simulink model "ADPSEStaF1LCLTr"  (R2018b)
settings: Solver=ode1  StartTime=0.0  StopTime=100  FixedStep=1/1000  RelTol=1e-3  AbsTol=1e-3  EnableMultiTasking=on
PostLoadFcn:
  | f_Simulink_figureplace
InitFcn:
  | ADPSEStaF1LCLTr_PreSim
values from neighbouring files (symbols this model uses):
  ar = 3    [ADPSEStaF1LCLTr_PreSim.m]
  beta = 0.01    [ADPSEStaF1LCLTr_PreSim.m]
  etaa1 = 2    [ADPSEStaF1LCLTr_PreSim.m]
  etaa2 = 0.0010    (= 0.001)    [ADPSEStaF1LCLTr_PreSim.m]
  etac1 = 0.001    [ADPSEStaF1LCLTr_PreSim.m]
  etac2 = 2    [ADPSEStaF1LCLTr_PreSim.m]
  F = 9    [ADPSEStaF1LCLTr_PreSim.m]
  freq = unifrnd(80,100,4,100)    [ADPSEStaF1LCLTr_PreSim.m]
  fs = 1000    [ADPSEStaF1LCLTr_PreSim.m]
  Gamma0 = 50*eye(L)    [ADPSEStaF1LCLTr_PreSim.m]
  GammaTheta = 1*eye(outlayer)    [ADPSEStaF1LCLTr_PreSim.m]
  k = 500    [ADPSEStaF1LCLTr_PreSim.m]
  kTheta = M*2    (= 20)    [ADPSEStaF1LCLTr_PreSim.m]
  m = 1    [ADPSEStaF1LCLTr_PreSim.m]
  M = 10    [ADPSEStaF1LCLTr_PreSim.m]
  model = 0    [ADPSEStaF1LCLTr_PreSim.m]
  MovePoints = 1    [ADPSEStaF1LCLTr_PreSim.m]
  n = 2    [ADPSEStaF1LCLTr_PreSim.m]
  Phase = unifrnd(0,2*pi,4,100)    [ADPSEStaF1LCLTr_PreSim.m]
  Q = [10 0 ; 0 10]    [ADPSEStaF1LCLTr_PreSim.m]
  R = 1    [ADPSEStaF1LCLTr_PreSim.m]
  s = 0.7    [ADPSEStaF1LCLTr_PreSim.m]
  theta0 = 0*ones(outlayer,n)    [ADPSEStaF1LCLTr_PreSim.m]
  v = 1    [ADPSEStaF1LCLTr_PreSim.m]
  WaH0 = 0.025*ones(L,1)    [ADPSEStaF1LCLTr_PreSim.m]
  WcH0 = 0.025*ones(L,1)    [ADPSEStaF1LCLTr_PreSim.m]
  x0 = [0; 0]    [ADPSEStaF1LCLTr_PreSim.m]
undefined symbols (not defined in the file or in its folder): g, outlayer
settings Model: Creator=rkamalapurkar  LastModifiedBy=rushik
settings SolverCC: AutoScaleAbsTol=off
settings DataIOCC: SaveFormat=Array  SaveOutput=off  DSMLogging=off  SaveTime=off  SignalLoggingName=ADPSEStaF1LCLTrData
settings OptimizationCC: ExpressionDepthLimit=2147483647  LifeSpan=inf  SimCompilerOptimization=on
settings DebuggingCC: UnderspecifiedInitializationDetection=Classic  MergeDetectMultiDrivingBlocksExec=none  SolverPrmCheckMsg=warning  FcnCallInpInsideContextMsg=warning  StateNameClashWarn=warning  SFUnexpectedBacktrackingDiag=warning  SFNoUnconditionalDefaultTransitionDiag=warning  SFExecutionAtInitializationDiag=none
settings HardwareCC: ProdBitPerPointer=32  ProdBitPerSizeT=32  ProdBitPerPtrDiffT=32  ProdLargestAtomicFloat=None  ProdIntDivRoundTo=Undefined  ProdEndianess=Unspecified  ProdWordSize=32  ProdHWDeviceType=32-bit Generic
settings ModelReferenceCC: PropagateSignalLabelsOutOfModel=off
settings SFSimCC: SimUseLocalCustomCode=off
settings RTWCC: RTWUseLocalCustomCode=off
settings CodeAppCC: StateflowObjectComments=on
settings GRTTargetCC: TargetLangStandard=C89/C90 (ANSI)  GeneratePreprocessorConditionals=Disable all  CombineOutputUpdateFcns=off  GRTInterface=on
settings ConfigComp: CovMetricSettings=dw  CovHtmlReporting=on  CovSaveCumulativeToWorkspaceVar=on  CovSaveSingleToWorkspaceVar=on  CovExternalEMLEnable=off  CovSFcnEnable=off

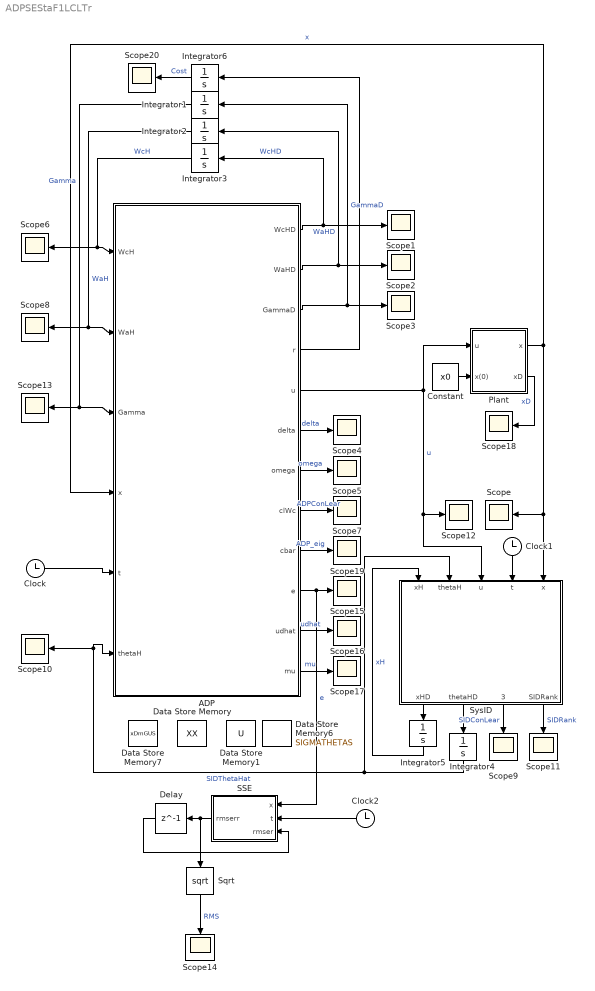
== system ADPSEStaF1LCLTr ==
  ADP : MATLAB Function  TreatAsAtomicUnit=on
  Clock : Clock
  Clock1 : Clock
  Clock2 : Clock
  Constant : Constant  Value=x0
  Data Store Memory : DataStoreMemory  DataStoreName=XX  InitialValue=zeros(n,F)  ShowAdditionalParam=off  OutDataTypeStr=double
  Data Store Memory1 : DataStoreMemory  DataStoreName=U  InitialValue=zeros(m,(F+1)/2)  ShowAdditionalParam=off  OutDataTypeStr=double
  Data Store Memory6 : DataStoreMemory  DataStoreName=SIGMATHETAS  InitialValue=zeros((outlayer),M)  ShowAdditionalParam=off  OutDataTypeStr=double
  Data Store Memory7 : DataStoreMemory  DataStoreName=xDmGUS  InitialValue=zeros(n,M)  ShowAdditionalParam=off  OutDataTypeStr=double
  Delay : Delay  DelayLength=1  InitialCondition=0
  Integrator1 : Integrator  InitialCondition=Gamma0
  Integrator2 : Integrator  InitialCondition=WaH0
  Integrator3 : Integrator  InitialCondition=WcH0
  Integrator4 : Integrator  InitialCondition=theta0
  Integrator5 : Integrator  InitialCondition=zeros(n,1)
  Integrator6 : Integrator
  Plant : Subsystem
  SSE : MATLAB Function  TreatAsAtomicUnit=on
  Scope{,1..20} (21 alike) : Scope
  Sqrt : Sqrt  SaturateOnIntegerOverflow=on
  SysID : MATLAB Function  TreatAsAtomicUnit=on
  wires:
  ADP/3(GammaD) -> Integrator1/1, Scope3/1  "GammaD"
  ADP/1(WcHD) -> Integrator3/1, Scope1/1  "WcHD"
  Integrator3/1 -> Scope6/1, ADP/1(WcH)  "WcH"
  ADP/2(WaHD) -> Integrator2/1, Scope2/1  "WaHD"
  Integrator2/1 -> Scope8/1, ADP/2(WaH)  "WaH"
  ADP/6(delta) -> Scope4/1  "delta"
  ADP/7(omega) -> Scope5/1  "omega"
  Integrator1/1 -> Scope13/1, ADP/3(Gamma)  "Gamma"
  Clock/1 -> ADP/5(t)
  ADP/5(u) -> Plant/1(u), SysID/3(u), Scope12/1  "u"
  ADP/8(clWc) -> Scope7/1  "ADPConLear"
  Integrator4/1 -> ADP/6(thetaH), Scope10/1, SysID/2(thetaH)  "SIDThetaHat"
  Plant/1(x) -> SysID/5(x), Scope/1, ADP/4(x)  "x"
  Constant/1 -> Plant/2(x(0))
  SysID/1(xHD) -> Integrator5/1
  Integrator5/1 -> SysID/1(xH)  "xH"
  SysID/4(SIDRank) -> Scope11/1  "SIDRank"
  SysID/3(SIDConLear) -> Scope9/1  "SIDConLear"
  SysID/2(thetaHD) -> Integrator4/1
  Clock1/1 -> SysID/4(t)
  ADP/10(e) -> SSE/1(x), Scope15/1  "e"
  ADP/11(udhat) -> Scope16/1  "udhat"
  ADP/12(mu) -> Scope17/1  "mu"
  Plant/2(xD) -> Scope18/1  "xD"
  ADP/9(cbar) -> Scope19/1  "ADP_eig"
  Clock2/1 -> SSE/2(t)
  SSE/1(rmserr) -> Sqrt/1, Delay/1
  Delay/1 -> SSE/3(rmser)
  Sqrt/1 -> Scope14/1  "RMS"
  ADP/4(r) -> Integrator6/1
  Integrator6/1 -> Scope20/1  "Cost"

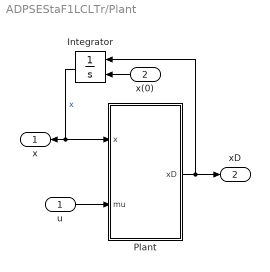
== system ADPSEStaF1LCLTr/Plant ==
  u : Inport
  x(0) : Inport  Port=2
  Integrator : Integrator  InitialConditionSource=external  InitialCondition=[1;1;0.0;0.0]
  Plant : MATLAB Function  TreatAsAtomicUnit=on
  x : Outport
  xD : Outport  Port=2
  wires:
  Plant/1(xD) -> Integrator/1, xD/1
  Integrator/1 -> Plant/1(x), x/1  "x"
  u/1 -> Plant/2(mu)
  x(0)/1 -> Integrator/2

== matlab function ADPSEStaF1LCLTr/SSE ==
  data: x input; t input; rmser input; rmserr output
function rmserr = fcn(x,t,rmser)
%#codegen

if t>90
    rmserr = rmser+(1/10000)*(norm(x))^2;
else
    rmserr = 0;
end

== matlab function ADPSEStaF1LCLTr/ADP ==
  settings: updateMethod=DISCRETE
  data: WcH input; WaH input; Gamma input; x input; t input; thetaH input; R parameter; Q parameter; etaa1 parameter; etaa2 parameter; etac1 parameter; v parameter; model parameter; WcHD output; WaHD output; GammaD output; r output; u output; delta output; omega output; clWc output; cbar output; etac2 parameter; beta parameter; n parameter; e output; udhat output; mu output; s parameter; MovePoints parameter; ar parameter; freq parameter; Phase parameter
function [WcHD,WaHD,GammaD,r,u,delta,omega,clWc,cbar,e,udhat,mu]=...
    control(WcH,WaH,Gamma,x,t,thetaH,R,Q,etaa1,etaa2,etac1,v,model,...
    etac2,beta,n,s,MovePoints,ar,freq,Phase)
%#codegen
% xd = [2*sin((1/2)*t); 2*cos((1/2)*t)+2*sin((1/2)*t)];
% if NormDyn == 1
%     a = norm(x0);
% else
%     a = 1;
% end
xd = (1/2)*[2*sin(t); 2*cos(t)+2*sin(t)];
hd = [xd(2)-xd(1); xd(2)-2*xd(1)];
e = x-xd;
Z = [e;xd];
%% Concurrent Learning
if model==1
    thetaH=[-1 -0.5; 1 0; 0 -0.5];
end
% nm=(y'*y+dbar)/(1+v2*(y'*y));
nm=1;
if MovePoints == 0
    temp=linspace(-3.0*s,3.0*s,3);
    [temp1, temp2, temp3, temp4] = ndgrid(temp,temp,temp,temp);
    XC=[temp1(:) temp2(:) temp3(:) temp4(:)]'; % matrix with columns as selected points
    N = length(temp)^(2*n); %Number of points
else
    N=1;
    XC=unifrnd(-ar*s*nm,ar*s*nm,2*n,N);
%     XC = ar*s*nm*ADPSEStaF1LCLTr_ExtTraj(t,freq,Phase);
end
clWc=zeros(size(WcH));
clWa=zeros(size(WaH));
CLmatrix=zeros(size(WcH,1),size(WcH,1));
CLGamma=zeros(size(Gamma));
parfor i=1:N
    Zi=Z+XC(:,i);
    ei=Zi(1:2,1);
    xdi=Zi(3:4,1);
    xi=ei+xdi;
    hdi = [xdi(2)-xdi(1);xdi(2)-2*xdi(1)];
    gi=[0; (cos(2*xi(1))+2)];
    gplusdi=[0 1/(cos(2*xdi(1))+2)];
    F1i = [-hdi+gi*gplusdi*hdi;hdi];
    [sigthi,~]=ADPSEStaF1LCLTr_SIDBasis(xi);
    [sigthdi,~]=ADPSEStaF1LCLTr_SIDBasis(xdi);
    Gi = [gi;zeros(size(gi))];
    [~,sig_pi,~]=ADPSEStaF1LCLTr_Basis(Zi,s,n);         
    mui=-0.5*(R\Gi')*sig_pi'*WaH;
    FTHi=[thetaH'*sigthi-gi*gplusdi*thetaH'*sigthdi;zeros(n,1)];
    omegai = sig_pi*(FTHi+F1i+Gi*mui);
%     rhoi=(1+v*omegai'*(Gamma)*omegai);
    rhoi=(1+v*(omegai'*omegai));
    ri = ei'*Q*ei + mui'*R*mui;
    deltai = WcH'*omegai + ri;
    clWc=clWc+Gamma*omegai*deltai/rhoi;
    Gsigmai = sig_pi*Gi*(R\Gi')*sig_pi';
    clWa=clWa+Gsigmai'*WaH*omegai'*WcH/(4*rhoi);
    CLmatrix=CLmatrix+omegai*omegai'/(N*rhoi);
    CLGamma=CLGamma+Gamma*(omegai*omegai'/rhoi^2)*Gamma;
end
clWc=-etac2*clWc/N;
clWa=etac2*clWa/N;
CLGamma=CLGamma/N;
cbar=real(min(svd(CLmatrix)));

%% ADP
g=[0; (cos(2*x(1))+2)];
gplusd=[0 1/(cos(2*xd(1))+2)];
F1 = [-hd+g*gplusd*hd;hd];
[sigth,~]=ADPSEStaF1LCLTr_SIDBasis(x);
[sigthd,~]=ADPSEStaF1LCLTr_SIDBasis(xd);
udhat = gplusd*(hd-thetaH'*sigthd);
G = [g;zeros(size(g))];
[~,sig_p,~]=ADPSEStaF1LCLTr_Basis(Z,s,n);         
mu=-0.5*(R\G')*sig_p'*WaH;
FTH=[thetaH'*sigth-g*gplusd*thetaH'*sigthd;zeros(n,1)];
omega = sig_p*(FTH+F1+G*mu);
Gsigma = sig_p*G*(R\G')*sig_p';
r = e'*Q*e + mu'*R*mu;
delta = WcH'*omega + r;
rho = (1+v*(omega'*omega));
WcHD = (-etac1*Gamma*omega*delta/rho+clWc);
GammaD = (beta*Gamma-Gamma*(omega*omega'/rho^2)*Gamma-CLGamma);
WaHD = etaa1*(WcH-WaH)...
    -(etaa2*WaH-etac1*Gsigma'*WaH*omega'*WcH/(4*rho))+clWa;
%% Controller
u = mu+udhat;

== matlab function ADPSEStaF1LCLTr/Plant/Plant ==
  data: xD output; x input; mu input
function xD = dynamics(x,mu)
%#codegen
F=[-x(1)+x(2) ;-0.5*x(1)-0.5*x(2)*(1-(cos(2*x(1))+2)^2)];
G=[0; (cos(2*x(1))+2)];
xD = F+G*mu;

== matlab function ADPSEStaF1LCLTr/SysID ==
  settings: updateMethod=DISCRETE
  data: xH input; xHD output; thetaH input; thetaHD output; u input; SIDConLear output; SIDRank output; t input; x input; k parameter; GammaTheta parameter; kTheta parameter; M parameter; XX data_store_memory; fs parameter; F parameter; g parameter; U data_store_memory; model parameter; SIGMATHETAS data_store_memory; xDmGUS data_store_memory
function [xHD,thetaHD,SIDConLear,SIDRank] = Control(xH,thetaH,u,t,x,k,...
    GammaTheta,kTheta,M,fs,F,g,model)
%#codegen
% This simulink block implements concurrent-learning based system
% identification using a Savitzky–Golay smoothing filter for state
% derivative computation. 
% fs: Sampling frequency
% M: number of stored data points
% F: Savitzky–Golay filter window length
% g: Savitzky–Golay filter differentiation matrix

global XX; % Data store memory for storing the values of x
global U; % Data store memory for storing the values of u
global SIGMATHETAS; % Data store for storing the values of sigth,
           % made of sigth matrices stacked in a row
global xDmGUS; % Data store memory for storing the values of xDot-G*u

%Dynamics
G=[0; (cos(2*x(1))+2)];

if model~=1
ite=round(t*fs)+1; % Current iteration number
xT = x-xH;

% Basis functions
[sigth,~]=ADPSEStaF1LCLTr_SIDBasis(x);

% At every time ite store the past F values of the state. Note that 
% Q*g(:,2)/(1/fs) gives the state derivative at ite-(F-1)/2
if ite<=F
    XX(:,ite)=x;
else
    XX = [XX(:,2:F) x];
end

% At every time ite store the past (F+1)/2 values of the control. Actually, 
% we only need the value of u at ite-(F-1)/2. However, I could not find a 
% way to store just that single value. Also, even if U is initialized as a 
% row vector, MATLAB seems to think its a column.
if ite<=(F+1)/2
    U(ite)=u;
else
    U = [U(2:(F+1)/2); u];
end

% The state derivative information is only available if ite>=F use
% singular value maximization algorithm to replace elements of SIGMATHETAS
% and XDmGUS with new data. At each time ite, the value of the 
% state at ite-(F-1)/2 can be found in XX(:,(F+1)/2)
index=0;
if ite>=F
    xj=XX(:,(F+1)/2);
    [sigthj,~]=ADPSEStaF1LCLTr_SIDBasis(xj);
    REGste1 = SIGMATHETAS*SIGMATHETAS'; % Compute Summation
    svd1=min(svd(REGste1));
    for i=1:M
         % Store existing data in a temporary variable
        SIGMATHETASte=SIGMATHETAS;
        % Replac i'th sigth matrix with sigthj
        SIGMATHETASte(:,i)=sigthj;
        REGste2 = SIGMATHETASte*SIGMATHETASte'; % Compute Summation
        svd2=min(svd(REGste2)); % Minimum singular value after replacement
        if svd1<svd2 % If replacement results in a higher singular value,
            index=i; % note the index of replacement and
            svd1=svd2; % keep searching for an even higher singular value.           
        end
    end
    
% At this point, index points to the matrix sigth in the stack 
% SIGMATHETAS which, when replaced with the new matrix sigthj,
% results in the highest singular value.
% If index=0, the new data point is discarded. Otherwise, the stack
% SIGMATHETAS, and correspondingly the stack xDmGUS is updated with the 
% new data point.
% Note that since there is a delay of (F-1)/2 for derivative computation,
% the "new" data point we are talking about is the one that was recorded 
% (F-1)/2 steps ago.
    if index ~= 0
        SIGMATHETAS(:,index)=sigthj;
        uj=U(1,1);
        xDj=XX*g(:,2)/(1/fs);
        Gj = [0; (cos(2*xj(1))+2)]; 
        xDmGUS(:,index)=xDj-Gj*uj;
    end
end

xHD = thetaH'*sigth + G*u + k*xT;

% Final computation for the concurrent learning-based component of the
% adaptive update law. The concurrent learning component is zero for the
% first F timesteps.
REGs = SIGMATHETAS*SIGMATHETAS'*(ite>=F);
SIDRank = min(svd(REGs)); % For plots
REG1s = SIGMATHETAS*xDmGUS'*(ite>=F);
SIDConLear = (REG1s-REGs*thetaH)/M;
thetaHD = (GammaTheta*sigth*xT' + kTheta*GammaTheta*SIDConLear);
else
SIDConLear = zeros(size(thetaH));
SIDRank = 0;
xHD = zeros(size(xH));    
thetaHD = zeros(size(thetaH));
end
